simulink model "quaternion_attitude_control_tracking"  (R2024b)
settings: Solver=VariableStepAuto  StartTime=0.0  StopTime=1200  MaxStep=0.2
values from neighbouring files (symbols this model uses):
  Cross_section_area = 0.01    [init_conditions.m]
  d = 0.8    [init_conditions.m]
  J = calculateInertiaTensor(mass, sideLength)    [init_conditions.m]
  k = 0.32    [init_conditions.m]
  mass = 1.33    [init_conditions.m]
  vec = [lat,long,alt]    [init_conditions.m]
undefined symbols (not defined in the file or in its folder): compute_drag
libraries: aerolibsatdyn x1, aerolibgravity2 x1
settings Model: VariantFading=off  LastModifiedBy=shavykashyap
settings SolverCC: ZeroCrossAlgorithm=Adaptive
settings DataIOCC: Refine=2
settings DebuggingCC: MaskedZcDiagnostic=none  IgnoredZcDiagnostic=none

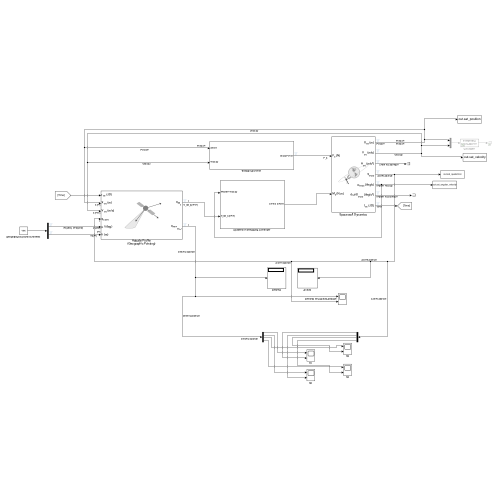
[thumbnail: Simulink's stored preview of the top-level diagram]
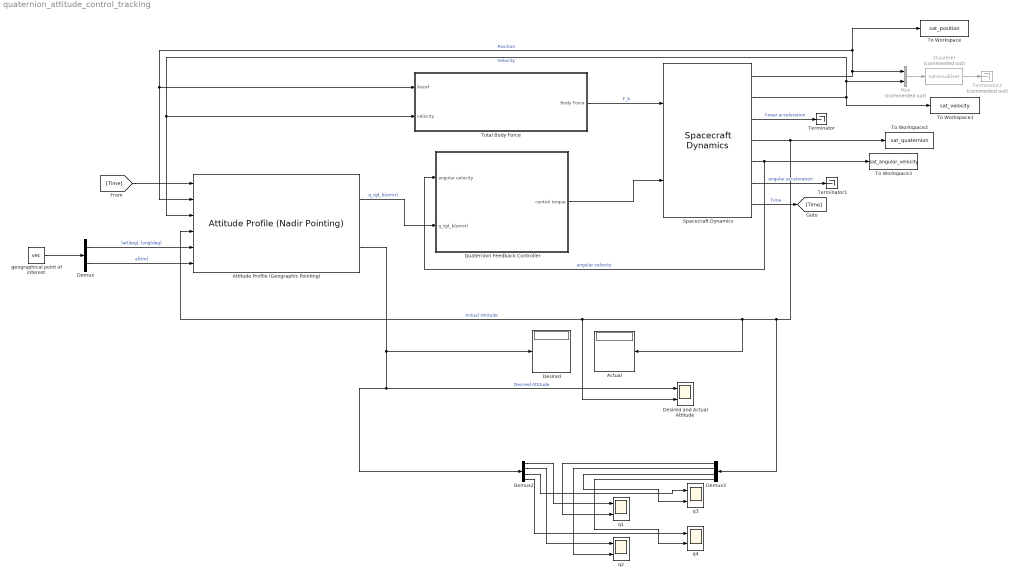
== system quaternion_attitude_control_tracking ==
  Actual : Display
  Attitude Profile (Geographic Pointing) : aerolibsatdyn/Attitude Profile (Nadir Pointing)  outputError=on  outputFinalAttitude=on  portFrame=ICRF  pointingMode=Point at LatLonAlt  celestialTarget=Sun  tunablePointing=off  primaryAlignmentSrc=Dialog  primaryAlignment=[0 0 1]  secondaryAlignmentSrc=Dialog  secondaryAlignment=[1 0 0]  constraintFrame=LVLH  primaryConstraintSrc=Dialog  primaryConstraint=[1 0 0]  secondaryConstraintSrc=Dialog  secondaryConstraint=[0 1 0]
      settings: LibrarySourceBlock=|
      | aerolibsatdyn/Attitude Profile
      | (Geographic Pointing)
  Demux : Demux  Outputs=2
  Demux2 : Demux
  Demux3 : Demux
  Desired : Display
  Desired and Actual Attitude : Scope  NumInputPorts=2
  Mux : Mux  Commented=on  Inputs=2
  "Quaternion Feedback Controller " : Subsystem
  Spacecraft Dynamics : SpacecraftDynamics  outputAccel=on  mass=mass  inertia=J  stateFormatNum=ICRF state vector  inertialPosition=initialPosition  inertialVelocity=initialVelocity  attitude=initialAttitude  attitudeRate=initialAngularVelocity  outputAngAccel=on  gravityModel=Oblate ellipsoid (J2)  useDrag=on  useSRP=on
  Terminator : Terminator
  Terminator1 : Terminator
  Terminator2 : Terminator  Commented=on
  To Workspace : ToWorkspace  VariableName=sat_position  SaveFormat=Timeseries  SampleTime=-1
  To Workspace1 : ToWorkspace  VariableName=sat_velocity  SaveFormat=Timeseries  SampleTime=-1
  To Workspace2 : ToWorkspace  VariableName=sat_quaternion  SaveFormat=Timeseries  SampleTime=-1
  To Workspace3 : ToWorkspace  VariableName=sat_angular_velocity  SaveFormat=Timeseries  SampleTime=-1
  "Total Body Force " : Subsystem
  VIsualiser : MATLABFcn  Commented=on  MATLABFcn=satvisualiser
  geographical point of interest : Constant  Value=vec
  q{1..4} (4 alike) : Scope  NumInputPorts=2
  wires:
  Spacecraft Dynamics/1 -> To Workspace/1, "Total Body Force "/1(Xecef), Attitude Profile (Geographic Pointing)/2, Mux/1  "Position"
  Spacecraft Dynamics/2 -> Mux/2, "Total Body Force "/2(velocity), Attitude Profile (Geographic Pointing)/3, To Workspace1/1  "Velocity"
  Spacecraft Dynamics/3 -> Terminator/1  "linear acceleration"
  Spacecraft Dynamics/4 -> To Workspace2/1, Demux3/1, Desired and Actual Attitude/2, Attitude Profile (Geographic Pointing)/4, Actual/1  "Actual Attitude"
  geographical point of interest/1 -> Demux/1
  Demux/1 -> Attitude Profile (Geographic Pointing)/5  "lat(deg), long(deg)"
  Demux/2 -> Attitude Profile (Geographic Pointing)/6  "alt(m)"
  Spacecraft Dynamics/6 -> Terminator1/1  "angular acceleration"
  Spacecraft Dynamics/7 -> [Time]  "Time"
  Attitude Profile (Geographic Pointing)/2 -> Demux2/1, Desired and Actual Attitude/1, Desired/1  "Desired Attitude"
  "Total Body Force "/1(Body Force) -> Spacecraft Dynamics/1  "F_b"
  [Time] -> Attitude Profile (Geographic Pointing)/1
  Demux2/1 -> q1/1
  Demux3/1 -> q1/2
  Demux2/2 -> q2/1
  Demux2/3 -> q3/1
  Demux2/4 -> q4/1
  Demux3/2 -> q2/2
  Demux3/3 -> q3/2
  Demux3/4 -> q4/2
  Spacecraft Dynamics/5 -> To Workspace3/1, "Quaternion Feedback Controller "/1(angular velocity)  "angular velocity"
  Attitude Profile (Geographic Pointing)/1 -> "Quaternion Feedback Controller "/2(q_tgt_b(error))  "q_tgt_b(error)"
  "Quaternion Feedback Controller "/1(control torque) -> Spacecraft Dynamics/2
  Mux/1 -> VIsualiser/1
  VIsualiser/1 -> Terminator2/1

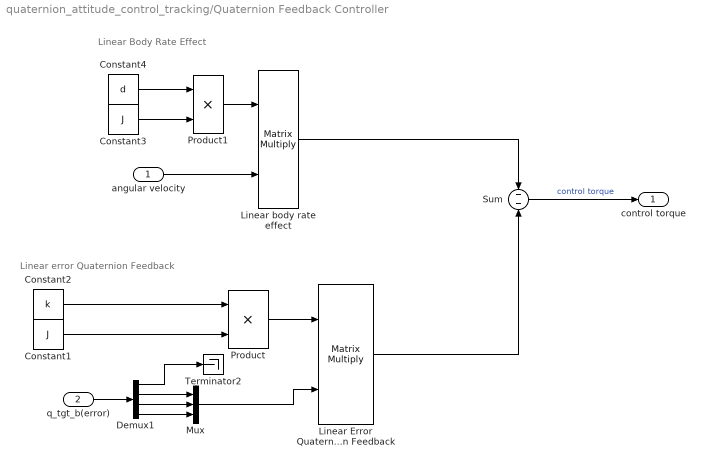
== system quaternion_attitude_control_tracking/Quaternion Feedback Controller  ==
  note: Linear error Quaternion Feedback
  note: Linear Body Rate Effect
  angular velocity : Inport
  q_tgt_b(error) : Inport  Port=2
  Constant1 : Constant  Value=J
  Constant2 : Constant  Value=k
  Constant3 : Constant  Value=J
  Constant4 : Constant  Value=d
  Demux1 : Demux
  Linear Error Quaternion Feedback : Product  Multiplication=Matrix(*)
  Linear body rate effect : Product  Multiplication=Matrix(*)
  Mux : Mux  Inputs=3
  Product : Product
  Product1 : Product
  Sum : Sum  Inputs=--
  Terminator2 : Terminator
  control torque : Outport
  wires:
  Linear body rate effect/1 -> Sum/1
  Mux/1 -> Linear Error Quaternion Feedback/2
  angular velocity/1 -> Linear body rate effect/2
  Demux1/1 -> Terminator2/1
  Constant1/1 -> Product/2
  Linear Error Quaternion Feedback/1 -> Sum/2
  Demux1/4 -> Mux/3
  Constant2/1 -> Product/1
  Demux1/2 -> Mux/1
  Demux1/3 -> Mux/2
  Constant3/1 -> Product1/2
  q_tgt_b(error)/1 -> Demux1/1
  Sum/1 -> control torque/1  "control torque"
  Constant4/1 -> Product1/1
  Product/1 -> Linear Error Quaternion Feedback/1
  Product1/1 -> Linear body rate effect/1

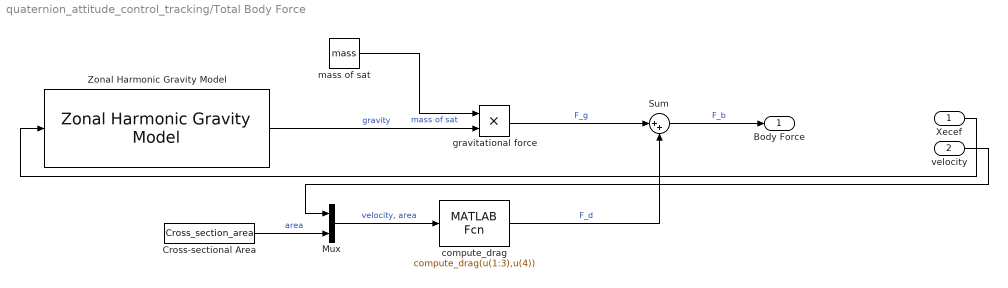
== system quaternion_attitude_control_tracking/Total Body Force  ==
  Xecef : Inport
  velocity : Inport  Port=2
  Cross-sectional Area : Constant  Value=Cross_section_area
  Mux : Mux  Inputs=2
  Sum : Sum  Inputs=|++
  Zonal Harmonic Gravity Model : aerolibgravity2/Zonal Harmonic Gravity Model  units=Metric (MKS)  degree=4  action=Warning  ptype=Earth  R=6378136.3  GM=398600441500000  jvalue=[1.0826269e-03 -2.5323000e-06 -1.6204000e-06]
  compute_drag : MATLABFcn  MATLABFcn=compute_drag(u(1:3),u(4))
  gravitational force : Product
  mass of sat : Constant  Value=mass
  Body Force : Outport
  wires:
  mass of sat/1 -> gravitational force/1  "mass of sat"
  compute_drag/1 -> Sum/2  "F_d"
  Mux/1 -> compute_drag/1  "velocity, area"
  Cross-sectional Area/1 -> Mux/2  "area"
  gravitational force/1 -> Sum/1  "F_g"
  Zonal Harmonic Gravity Model/1 -> gravitational force/2  "gravity"
  Xecef/1 -> Zonal Harmonic Gravity Model/1
  Sum/1 -> Body Force/1  "F_b"
  velocity/1 -> Mux/1
